simulink model "PandO"  (R2017b)
settings: Solver=VariableStepAuto  StartTime=0.0  StopTime=10.0  RelTol=1e-3
settings Model: Creator=SeanP  LastModifiedBy=SeanP

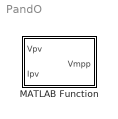
== system PandO ==
  MATLAB Function : MATLAB Function  TreatAsAtomicUnit=on

== matlab function PandO/MATLAB Function ==
  data: Vpv input; Vmpp output; Ipv input
function Vmpp = PandO(Vpv,Ipv)

persistent Vmpp_prev Vpv_prev Ppv_prev

%initialize variables if first pass
if isEmpty(Vmpp_prev)
    Vmpp_prev = 2409 .* 5; %set initial guess to Datasheet's MPP of 2409mV times 5 cells on center panel
    Vpv_prev = 2409 .* 5; %set inital voltage to assume we are already at MPP
    Ppv_prev = 2409 .* 5 .* .505; %set inital power to power at mpp from datasheet.
end

V_increment = 1; %increment Vmpp in steps of 1mV per pass.

%calculate measured power
Ppv = Vpv * Ipv;

%decide whether to increment or decrement. 
if (Ppv-Ppv_prev) ~= 0
    if (Ppv-Ppv_prev) > 0
        if (Vpv-Vpv_prev) > 0
            Vmpp = Vmpp_prev - V_increment;
        else
            Vmpp = Vmpp_prev + V_increment;
        end
    else
        if (Vpv-Vpv_prev) > 0
            Vmpp = Vmpp_prev + V_increment;
        else
            Vmpp = Vmpp_prev + V_increment;
        end
    end
else
    Vmpp = Vmpp_prev;
end

Vpv_prev = Vpv;
Ppv_prev = Ppv;
Vmpp_prev = Vmpp;
